simulink model "robot3_pdG_Cartasian"  (R2023b)
settings: Solver=VariableStepAuto  StartTime=0.0  StopTime=2*pi  RelTol=1e-3
undefined symbols (not defined in the file or in its folder): Cartesian_trajectory, Coriolis3, Dinv3, Forward_kin3, Gravity3, Jacobian3, JT3
settings Model: Creator=사용자  LastModifiedBy=사용자

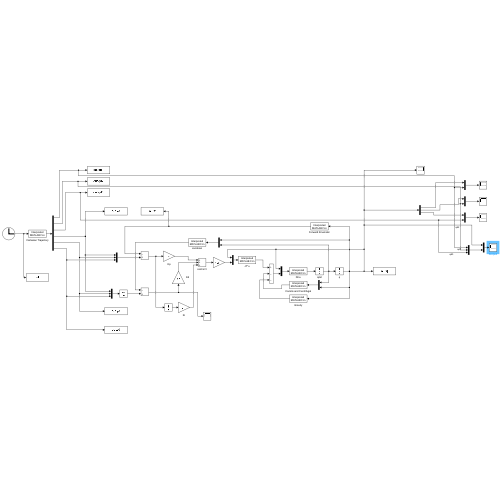
[thumbnail: Simulink's stored preview of the top-level diagram]
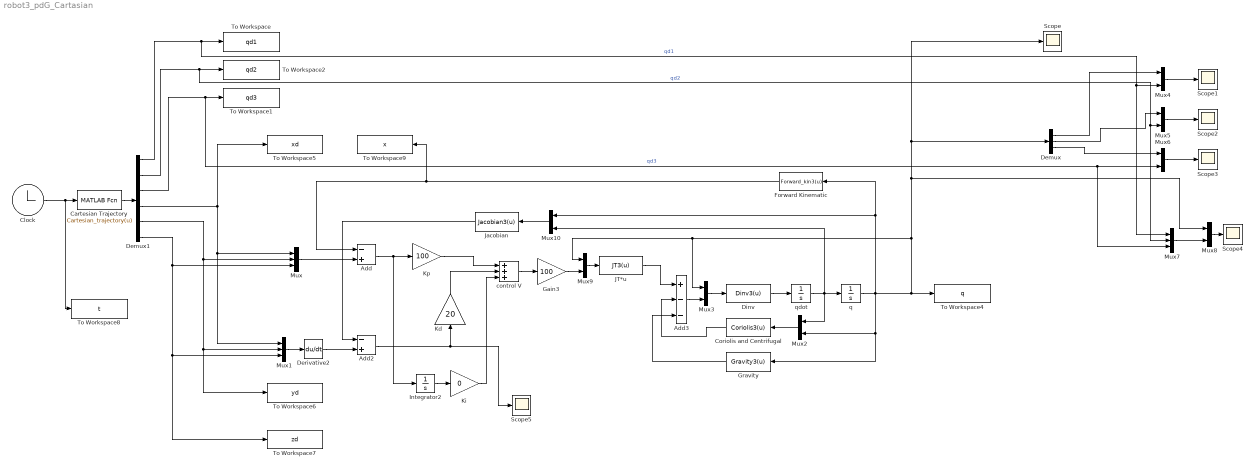
== system robot3_pdG_Cartasian ==
  Add : Sum  Inputs=-+
  Add2 : Sum  Inputs=-+
  Add3 : Sum  Inputs=+--
  Cartesian Trajectory : MATLABFcn  MATLABFcn=Cartesian_trajectory(u)  OutputDimensions=6  Output1D=off
  Clock : Clock
  Coriolis and Centrifugal : MATLABFcn  MATLABFcn=Coriolis3(u)  OutputDimensions=3  Output1D=off
  Demux : Demux  Outputs=3
  Demux1 : Demux  Outputs=6
  Derivative2 : Derivative
  Dinv : MATLABFcn  MATLABFcn=Dinv3(u)  OutputDimensions=3  Output1D=off
  Forward Kinematic : MATLABFcn  MATLABFcn=Forward_kin3(u)  OutputDimensions=3  Output1D=off
  Gain3 : Gain  Gain=100
  Gravity : MATLABFcn  MATLABFcn=Gravity3(u)  OutputDimensions=3  Output1D=off
  Integrator2 : Integrator  InitialCondition=[0.408;0.408;0.53];
  JT*u : MATLABFcn  MATLABFcn=JT3(u)  OutputDimensions=3  Output1D=off
  Jacobian : MATLABFcn  MATLABFcn=Jacobian3(u)  OutputDimensions=3  Output1D=off
  Kd : Gain  Gain=20
  Ki : Gain  Gain=0
  Kp : Gain  Gain=100
  Mux : Mux  Inputs=3
  Mux1 : Mux  Inputs=3
  Mux{2..6,8..10} (8 alike) : Mux  Inputs=2
  Mux7 : Mux  Inputs=3
  Scope{,1..5} (6 alike) : Scope
  To Workspace : ToWorkspace  VariableName=qd1  SaveFormat=Timeseries  SampleTime=0.001
  To Workspace1 : ToWorkspace  VariableName=qd3  SaveFormat=Timeseries  SampleTime=0.001
  To Workspace2 : ToWorkspace  VariableName=qd2  SaveFormat=Timeseries  SampleTime=0.001
  To Workspace4 : ToWorkspace  VariableName=q  SaveFormat=Timeseries  SampleTime=0.001
  To Workspace5 : ToWorkspace  VariableName=xd  SampleTime=0.001
  To Workspace6 : ToWorkspace  VariableName=yd  SampleTime=0.001
  To Workspace7 : ToWorkspace  VariableName=zd  SampleTime=0.001
  To Workspace8 : ToWorkspace  VariableName=t  SaveFormat=Timeseries  SampleTime=0.001
  To Workspace9 : ToWorkspace  VariableName=x  SampleTime=0.001
  control V : Sum  Inputs=+++
  q : Integrator  InitialCondition=[0.9587;0.7246;-1.1694]
  qdot : Integrator  InitialCondition=[0;0;0];
  wires:
  Add2/1 -> Scope5/1, Kd/1
  Kp/1 -> control V/1
  Kd/1 -> control V/2
  Add/1 -> Kp/1, Integrator2/1
  Add3/1 -> Mux3/2
  Mux3/1 -> Dinv/1
  Dinv/1 -> qdot/1
  Mux2/1 -> Coriolis and Centrifugal/1
  qdot/1 -> Mux10/2, Mux2/1, q/1
  Coriolis and Centrifugal/1 -> Add3/2
  Gravity/1 -> Add3/3
  q/1 -> Scope/1, Demux/1, Mux8/1, Mux3/1, Mux9/1, To Workspace4/1, Mux10/1, Forward Kinematic/1, Gravity/1, Mux2/2
  Mux4/1 -> Scope1/1
  Mux5/1 -> Scope2/1
  Mux6/1 -> Scope3/1
  Demux/1 -> Mux4/1
  Demux/2 -> Mux5/1
  Demux/3 -> Mux6/1
  Mux7/1 -> Mux8/2
  Mux8/1 -> Scope4/1
  Cartesian Trajectory/1 -> Demux1/1
  Demux1/1 -> Mux7/1, Mux4/2, To Workspace/1  "qd1"
  Demux1/2 -> Mux7/2, Mux5/2, To Workspace2/1  "qd2"
  Demux1/3 -> Mux7/3, Mux6/2, To Workspace1/1  "qd3"
  Demux1/4 -> Mux/1, Mux1/1, To Workspace5/1
  Demux1/5 -> Mux1/2, To Workspace6/1, Mux/2
  Demux1/6 -> To Workspace7/1, Mux1/3, Mux/3
  Mux1/1 -> Derivative2/1
  Clock/1 -> To Workspace8/1, Cartesian Trajectory/1
  Mux/1 -> Add/2
  Derivative2/1 -> Add2/2
  Forward Kinematic/1 -> To Workspace9/1, Add/1
  Integrator2/1 -> Ki/1
  Ki/1 -> control V/3
  Jacobian/1 -> Add2/1
  control V/1 -> Gain3/1
  Gain3/1 -> Mux9/2
  Mux9/1 -> JT*u/1
  JT*u/1 -> Add3/1
  Mux10/1 -> Jacobian/1
